simulink model "Full_Model_2"  (R2018b)
settings: Solver=VariableStepAuto  StartTime=0.0  StopTime=.25  RelTol=1e-3
InitFcn:
  | Robot_Body_Constants
values from neighbouring files (symbols this model uses):
  robot_mass = 0.743    [Robot_Body_Constants.m]
  robot_radius = 0.0789    [Robot_Body_Constants.m]
libraries: powerlib x14, simulink x1, peBldcCurrentController x1
settings Model: Creator=Zach  LastModifiedBy=Zach

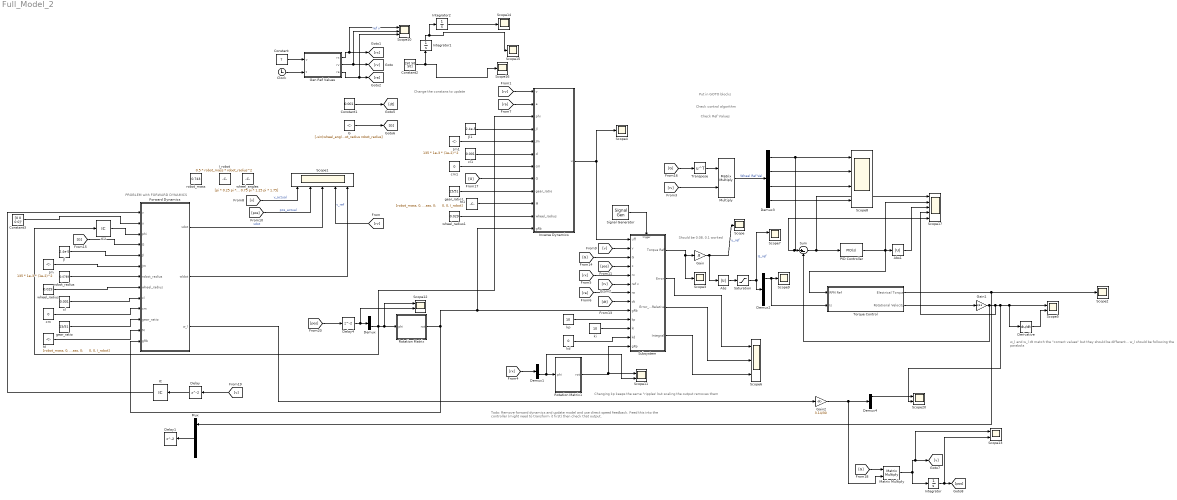
== system Full_Model_2 ==
  note: PROBLEM with FORWARD DYNAMICS
  note: w_l and w_l dt match the "correct values" but they should be different... w_l should be following the parabola
  note: Change the constans to update
  note: Todo: Remove forward dynamics and update model and use direct speed feedback. Feed this into the controller (might need to transform it first) then check that output.
  note: Should be 0.08, 0.1 worked
  note: Changing kp keeps the same "ripples' but scaling the output removes them
  note: Check Ref Values
  note: Check control algorithm
  note: Put in GOTO blocks
  Abs : Abs
  Abs1 : Abs
  Clock : Clock
  Constant : Constant  Value=7
  Constant1 : Constant  Value=0.001
  Constant2 : Constant  Value=[50 50 50]
  Constant3 : Constant  Value=[0 0 0 0]'
  Delay : Delay
  Delay1 : Delay
  Delay4 : Delay
  Demux : Demux  Outputs=3
  Demux1 : Demux  Outputs=3
  Demux2 : Demux
  Demux3 : Demux
  Demux4 : Demux
  Derivative : Derivative
  Forward Dynamics : MATLAB Function  TreatAsAtomicUnit=on
  G : Constant  Value=|
      | [-sin(wheel_angles(1)) -sin(wheel_angles(2)) -sin(wheel_angles(3)) -sin(wheel_angles(4));
      |      cos(wheel_angles(1)) cos(wheel_angles(2)) cos(wheel_angles(3)) cos(wheel_angles(4));
      |      robot_radius robot_radius robot_radius robot_radius]
  Gain : Gain  Gain=.8
  Gain1 : Gain  Gain=1/9.5
  Gain2 : Gain  Gain=3.14/30
  Gen Ref Values : MATLAB Function  TreatAsAtomicUnit=on
  IC : InitialCondition  Value=[0 0 0]'
  IC2 : InitialCondition  Value=0
  I_robot : Constant  Value=0.5 * robot_mass * robot_radius^2
  Integrator : Integrator
  Integrator1 : Integrator
  Integrator2 : Integrator
  Inverse Dynamics : MATLAB Function  TreatAsAtomicUnit=on
  Jl : Constant  Value=2.4e-5
  Jl1 : Constant  Value=2.4e-5
  Jm : Constant  Value=135 * 1e-3 * (1e-2)^2
  Jm1 : Constant  Value=135 * 1e-3 * (1e-2)^2
  M : Constant  Value=|
      | [robot_mass, 0, 0;
      |      0, robot_mass, 0;
      |      0, 0, I_robot]
  M1 : Constant  Value=|
      | [robot_mass, 0, 0;
      |      0, robot_mass, 0;
      |      0, 0, I_robot]
  Matrix Multiply : Product  Multiplication=Matrix(*)
  Multiply : Product  Multiplication=Matrix(*)
  Mux : Mux
  PID Controller : simulink/Continuous/PID Controller  Controller=PID  Form=Parallel  TimeDomain=Continuous-time  SampleTime=-1  IntegratorMethod=Forward Euler  FilterMethod=Forward Euler  ControllerParametersSource=internal  P=10  I=10  D=0  UseFilter=on  N=100  TunerSelectOption=Transfer Function Based (PID Tuner App)  InitialConditionSource=internal  InitialConditionForIntegrator=0  InitialConditionForFilter=0  DifferentiatorICPrevScaledInput=0  ExternalReset=none  TrackingMode=off  Kt=1  LimitOutput=on  UpperSaturationLimit=40  LowerSaturationLimit=-40  LinearizeAsGain=on  AntiWindupMode=none  Kb=1  POutMin=[]  POutMax=[]  IOutMin=[]  IOutMax=[]  DOutMin=[]  DOutMax=[]  NOutMin=[]  NOutMax=[]  SumOutMin=[]  SumOutMax=[]  SaturationOutMin=[]  SaturationOutMax=[]  PParamMin=[]  PParamMax=[]  IParamMin=[]  IParamMax=[]  DParamMin=[]  DParamMax=[]  NParamMin=[]  NParamMax=[]  KbParamMin=[]  KbParamMax=[]  KtParamMin=[]  KtParamMax=[]  KbOutMin=[]  KbOutMax=[]  KtOutMin=[]  KtOutMax=[]  IntegratorOutMin=[]  IntegratorOutMax=[]  FilterOutMin=[]  FilterOutMax=[]  SumI1OutMin=[]  SumI1OutMax=[]  SumI2OutMin=[]  SumI2OutMax=[]  SumI3OutMin=[]  SumI3OutMax=[]  SumI4OutMin=[]  SumI4OutMax=[]  SumDOutMin=[]  SumDOutMax=[]  DifferentiatorOutMin=[]  DifferentiatorOutMax=[]  FilterDiffOutCoefMin=[]  FilterDiffOutCoefMax=[]  ReciprocalOutMin=[]  ReciprocalOutMax=[]  SumDenOutMin=[]  SumDenOutMax=[]  SumNumOutMin=[]  SumNumOutMax=[]  DivideOutMin=[]  DivideOutMax=[]  IntegratorContinuousStateAttributes=''  IntegratorStateMustResolveToSignalObject=off  IntegratorRTWStateStorageClass=Auto  FilterContinuousStateAttributes=''  FilterStateMustResolveToSignalObject=off  FilterRTWStateStorageClass=Auto  ParallelPVariant=InternalParameters  IdealPVariant=Disabled  IVariant=InternalParameters  DVariant=InternalParameters  IntegratorVariant=Continuous  SatVariant=Enabled  AWVariant=Passthrough  PCopyVariant=Disabled  TRVariant=Disabled  FdbkBlocksVariant=Forward  IdealPFdbkVariant=Disabled  SatFdbkVariant=Disabled  DerivativeFilterVariant=ContFilter  NVariant=InternalParameters  NCopyVariant=Disabled  FilterICVariant=InternalICsFilter  IntegratorICVariant=InternalICs  ExternalResetVariant=Disabled  TRSumVariant=Passthrough  SumFdbkVariant=Disabled  SumVariant=Sum_PID
  Rotation Matrix : MATLAB Function  TreatAsAtomicUnit=on
  Rotation Matrix1 : MATLAB Function  TreatAsAtomicUnit=on
  Saturation : Saturate  UpperLimit=40  LowerLimit=-40
  Scope{,2..4,9,14..16} (8 alike) : Scope
  Scope1 : Scope  NumInputPorts=5
  Scope10 : Scope  NumInputPorts=3
  Scope{5,7,11..13,20} (6 alike) : Scope  NumInputPorts=2
  Scope17 : Scope  NumInputPorts=5
  Scope6 : Scope  NumInputPorts=3
  Scope8 : Scope  NumInputPorts=4
  Signal Generator : SignalGenerator  WaveForm=square  Frequency=300  Units=rad/sec
  Subsystem : Subsystem
  Sum : Sum  Inputs=|+-
  Torque Control : Subsystem
  Transpose : Math  Operator=transpose  SaturateOnIntegerOverflow=on
  cl : Constant  Value=0.001
  cl1 : Constant  Value=0.001
  cm : Constant  Value=0
  cm1 : Constant  Value=0
  gear_ratio : Constant  Value=15/51
  gear_ratio1 : Constant  Value=15/51
  kd : Constant  Value=0
  ki : Constant  Value=10
  kp : Constant  Value=10
  robot_mass : Constant  Value=0.743
  robot_radius : Constant  Value=0.0789
  wheel_angles : Constant  Value=[pi * 0.25 pi * 0.75 pi * 1.25 pi * 1.75]
  wheel_radius : Constant  Value=0.029
  wheel_radius1 : Constant  Value=0.029
  wires:
  Delay4/1 -> Scope12/2, Demux/1
  Delay/1 -> IC/1
  IC2/1 -> Forward Dynamics/3(phi)
  Clock/1 -> Gen Ref Values/2(t)
  cl1/1 -> Inverse Dynamics/6(cl)
  gear_ratio/1 -> Forward Dynamics/11(gear_ratio)
  Jm1/1 -> Inverse Dynamics/5(Jm)
  Jl1/1 -> Inverse Dynamics/4(Jl)
  Jl/1 -> Forward Dynamics/5(Jl)
  gear_ratio1/1 -> Inverse Dynamics/9(gear_ratio)
  Gain/1 -> Scope/1, Abs/1  "u_ref"
  Constant1/1 -> [dt]
  M/1 -> Forward Dynamics/12(M)
  Constant/1 -> Gen Ref Values/1(v)
  Rotation Matrix/1(rot) -> Forward Dynamics/13(gRb), Inverse Dynamics/12(gRb), Subsystem/9(gRb)
  Torque Control/1(Electrical Torque) -> Mux/1, Scope2/1
  wheel_radius1/1 -> Inverse Dynamics/11(wheel_radius)
  G/1 -> [G]
  IC/1 -> Forward Dynamics/1(v)
  cl/1 -> Forward Dynamics/9(cl)
  Forward Dynamics/1(vdot) -> Scope1/3  "vdot"
  M1/1 -> Inverse Dynamics/10(M)
  robot_radius/1 -> Forward Dynamics/7(robot_radius)
  cm1/1 -> Inverse Dynamics/7(cm)
  wheel_radius/1 -> Forward Dynamics/8(wheel_radius)
  cm/1 -> Forward Dynamics/10(cm)
  Inverse Dynamics/1(u) -> Subsystem/1(uff), Scope4/1
  Jm/1 -> Forward Dynamics/6(Jm)
  Demux3/2 -> Scope8/2
  Demux3/3 -> Scope8/3
  Demux3/4 -> Scope8/4
  Multiply/1 -> Demux3/1  "Wheel Ref Vel"
  Transpose/1 -> Multiply/1
  Subsystem/1(Torque Ref) -> Scope3/1, Gain/1
  kp/1 -> Subsystem/10(kp)
  ki/1 -> Subsystem/11(ki)
  kd/1 -> Subsystem/12(kd)
  Rotation Matrix1/1(rot) -> Scope11/1, Subsystem/13(gRp)
  Subsystem/2(Error) -> Scope6/1
  Subsystem/3(Error_Path_Relative) -> Scope6/2
  Subsystem/4(Integral) -> Scope6/3
  Signal Generator/1 -> Subsystem/Trigger
  [rv] -> Scope1/4  "v_ref"
  [rv] -> Inverse Dynamics/1(v)
  [rv] -> Subsystem/6(ref v)
  [rv] -> Multiply/2
  [rx] -> Demux1/1
  [rx] -> Subsystem/5(rx)
  [ra] -> Subsystem/7(ra)
  [ra] -> Inverse Dynamics/2(a)
  [v] -> Scope1/1  "v_actual"
  [v] -> Subsystem/2(v)
  [pos] -> Scope1/2  "pos_actual"
  [pos] -> Subsystem/4(x)
  [dt] -> Subsystem/8(dt)
  [G] -> Subsystem/3(G)
  [G] -> Forward Dynamics/4(G)
  [G] -> Transpose/1
  [G] -> Inverse Dynamics/8(G)
  Forward Dynamics/2(wldot) -> Scope1/5
  Abs/1 -> Saturation/1
  Demux2/1 -> Torque Control/2(Is), Scope9/1
  Gain1/1 -> Scope20/2, Derivative/1, Scope5/1, Scope17/4, Sum/2
  Demux/3 -> Inverse Dynamics/3(phi), Scope12/1, Rotation Matrix/1(phi), IC2/1
  Demux1/3 -> Scope11/2, Rotation Matrix1/1(phi)
  Saturation/1 -> Demux2/1, Scope7/1  "Is_ref"
  Gain2/1 -> Matrix Multiply/2, Demux4/1
  [G] -> Matrix Multiply/1
  Matrix Multiply/1 -> Integrator/1, Scope13/1, [v]
  Integrator/1 -> Scope13/2, [pos]
  [v] -> Delay/1
  [pos] -> Delay4/1
  Constant2/1 -> Integrator1/1, Scope16/1
  Integrator1/1 -> Scope15/1, Integrator2/1
  Integrator2/1 -> Scope14/1
  PID Controller/1 -> Abs1/1, Torque Control/1(RPM Ref), Scope17/2
  Abs1/1 -> Scope17/3
  Forward Dynamics/3(w_l) -> Gain2/1
  Demux4/1 -> Scope20/1
  Demux3/1 -> Scope8/1, Scope17/5, Sum/1
  Gen Ref Values/2(rv) -> Scope10/2, [rv]  "ref v"
  Gen Ref Values/1(rx) -> Scope10/1, [rx]
  Gen Ref Values/3(ra) -> Scope10/3, [ra]
  Sum/1 -> PID Controller/1, Scope17/1
  Torque Control/2(Rotational Velocity) -> Gain1/1
  Mux/1 -> Delay1/1
  Derivative/1 -> Scope5/2
  Constant3/1 -> Forward Dynamics/2(u)

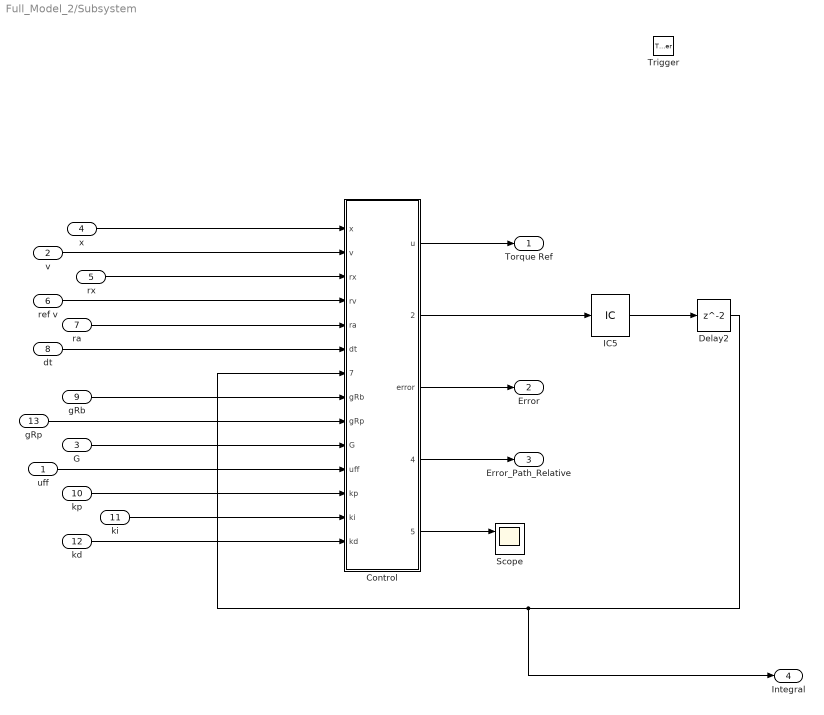
== system Full_Model_2/Subsystem ==
  uff : Inport
  v : Inport  Port=2
  G : Inport  Port=3
  x : Inport  Port=4
  rx : Inport  Port=5
  ref v : Inport  Port=6
  ra : Inport  Port=7
  dt : Inport  Port=8
  gRb : Inport  Port=9
  kp : Inport  Port=10
  ki : Inport  Port=11
  kd : Inport  Port=12
  gRp : Inport  Port=13
  Trigger : TriggerPort  VariantControl=Variant  PortDimensions=1
  Control : MATLAB Function  TreatAsAtomicUnit=on
  Delay2 : Delay
  IC5 : InitialCondition  Value=[0 0 0]
  Scope : Scope  NumInputPorts=2
  Torque Ref : Outport
  Error : Outport  Port=2
  Error_Path_Relative : Outport  Port=3
  Integral : Outport  Port=4
  wires:
  Delay2/1 -> Integral/1, Control/7("integral ")
  uff/1 -> Control/11(uff)
  Control/2(integral) -> IC5/1
  IC5/1 -> Delay2/1
  G/1 -> Control/10(G)
  Control/1(u) -> Torque Ref/1
  rx/1 -> Control/3(rx)
  gRb/1 -> Control/8(gRb)
  ki/1 -> Control/13(ki)
  gRp/1 -> Control/9(gRp)
  kd/1 -> Control/14(kd)
  x/1 -> Control/1(x)
  Control/3(error) -> Error/1
  ra/1 -> Control/5(ra)
  Control/4(error_path_relative) -> Error_Path_Relative/1
  dt/1 -> Control/6(dt)
  ref v/1 -> Control/4(rv)
  v/1 -> Control/2(v)
  kp/1 -> Control/12(kp)
  Control/5(wheel_ref) -> Scope/1

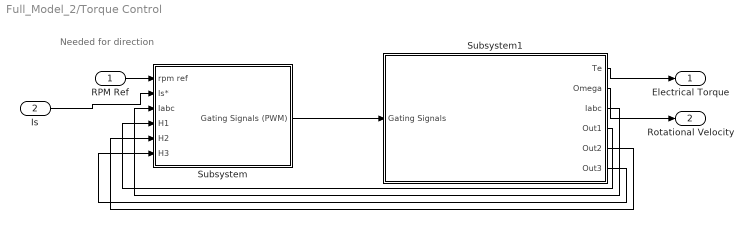
== system Full_Model_2/Torque Control ==
  note: Needed for direction
  RPM Ref : Inport
  Is : Inport  Port=2
  Subsystem : Subsystem
  Subsystem1 : Subsystem
  Electrical Torque : Outport
  Rotational Velocity : Outport  Port=2
  wires:
  Subsystem/1(Gating Signals (PWM)) -> Subsystem1/1(Gating Signals)
  RPM Ref/1 -> Subsystem/1(rpm ref)
  Is/1 -> Subsystem/2(Is*)
  Subsystem1/2(Omega) -> Rotational Velocity/1
  Subsystem1/1(Te) -> Electrical Torque/1
  Subsystem1/3(Iabc) -> Subsystem/3(Iabc)
  Subsystem1/4(Out1) -> Subsystem/4(H1)
  Subsystem1/5(Out2) -> Subsystem/5(H2)
  Subsystem1/6(Out3) -> Subsystem/6(H3)

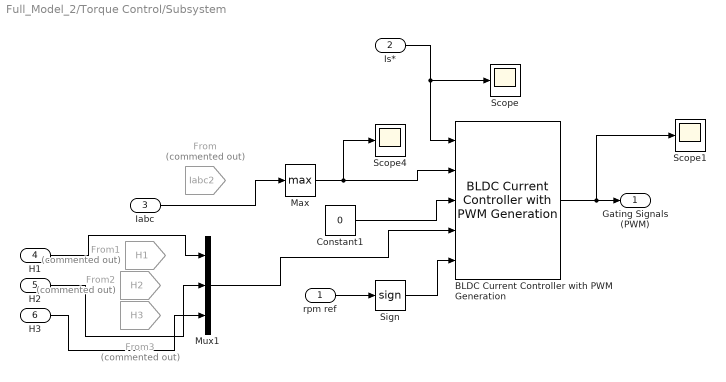
== system Full_Model_2/Torque Control/Subsystem ==
  rpm ref : Inport
  Is* : Inport  Port=2
  Iabc : Inport  Port=3
  H1 : Inport  Port=4
  H2 : Inport  Port=5
  H3 : Inport  Port=6
  BLDC Current Controller with PWM Generation : peBldcCurrentController/BLDC Current Controller with PWM Generation  Kp=40  Ki=10  Kaw=100  Ts=-1  Tsd=0.001  ActZC=off  CarrCount=Up  Tper=.0001  Tfundamental=.00001
  Constant1 : Constant  Value=0
  From : From  Commented=on  GotoTag=Iabc2  TagVisibility=global
  From1 : From  Commented=on  GotoTag=H1  TagVisibility=global
  From2 : From  Commented=on  GotoTag=H2  TagVisibility=global
  From3 : From  Commented=on  GotoTag=H3  TagVisibility=global
  Max : MinMax  Function=max
  Mux1 : Mux  Inputs=3
  Scope : Scope
  Scope1 : Scope
  Scope4 : Scope
  Sign : Signum
  Gating Signals (PWM) : Outport
  wires:
  rpm ref/1 -> Sign/1
  Mux1/1 -> BLDC Current Controller with PWM Generation/4
  Sign/1 -> BLDC Current Controller with PWM Generation/5
  Constant1/1 -> BLDC Current Controller with PWM Generation/3
  Max/1 -> BLDC Current Controller with PWM Generation/2, Scope4/1
  BLDC Current Controller with PWM Generation/1 -> Scope1/1, Gating Signals (PWM)/1
  Is*/1 -> Scope/1, BLDC Current Controller with PWM Generation/1
  Iabc/1 -> Max/1
  H1/1 -> Mux1/1
  H2/1 -> Mux1/2
  H3/1 -> Mux1/3

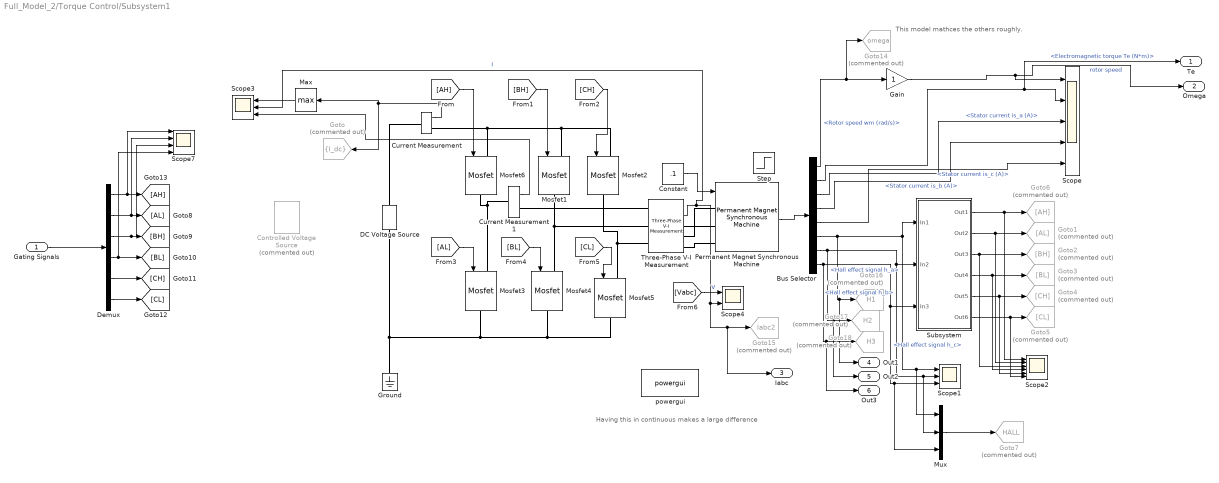
== system Full_Model_2/Torque Control/Subsystem1 ==
  note: This model mathces the others roughly.
  note: Having this in continuous makes a large difference
  Gating Signals : Inport
  Bus Selector : BusSelector  OutputSignals=Rotor speed wm (rad/s),Electromagnetic torque Te (N*m),Stator current is_a (A),Stator current is_b (A),Stator current is_c (A),Hall effect signal h_a,Hall effect signal h_b,Hall effect signal h_c
  Constant : Constant  Value=.1
  Controlled Voltage Source : powerlib/Electrical Sources/Controlled Voltage Source  Commented=on  Initialize=off  Source_Type=DC  Amplitude=24  Phase=0  Frequency=0  Measurements=Voltage
  Current Measurement : powerlib/Measurements/Current Measurement  PhasorSimulation=off  OutputType=Magnitude  PSBequivalent=0
  Current Measurement1 : powerlib/Measurements/Current Measurement  PhasorSimulation=off  OutputType=Complex  PSBequivalent=0
  DC Voltage Source : powerlib/Electrical Sources/DC Voltage Source  Amplitude=24  Measurements=None
  Demux : Demux  Outputs=6
  Gain : Gain
  Goto : Goto  Commented=on  GotoTag=I_dc  TagVisibility=scoped
  Goto1 : Goto  Commented=on  GotoTag=AL
  Goto14 : Goto  Commented=on  GotoTag=omega  TagVisibility=global
  Goto15 : Goto  Commented=on  GotoTag=Iabc2  TagVisibility=global
  Goto16 : Goto  Commented=on  GotoTag=H1  TagVisibility=global
  Goto17 : Goto  Commented=on  GotoTag=H2  TagVisibility=global
  Goto18 : Goto  Commented=on  GotoTag=H3  TagVisibility=global
  Goto2 : Goto  Commented=on  GotoTag=BH
  Goto3 : Goto  Commented=on  GotoTag=BL
  Goto4 : Goto  Commented=on  GotoTag=CH
  Goto5 : Goto  Commented=on  GotoTag=CL
  Goto6 : Goto  Commented=on  GotoTag=AH
  Goto7 : Goto  Commented=on  GotoTag=HALL  TagVisibility=global
  Ground : powerlib/Elements/Ground  LConnTagsString=a
  Max : MinMax  Function=max
  Mosfet{1..6} (6 alike) : powerlib/Power Electronics/Mosfet  Ron=0.1  Lon=0  Rd=0.01  Vfd=0  IC=0  Rs=1e5  Cs=inf  Measurements=off
  Mux : Mux  Inputs=3
  Permanent Magnet Synchronous Machine : powerlib/Machines/Permanent Magnet Synchronous Machine  NbPhases=3  FluxDistribution=Trapezoidal  RotorType=Round  MechanicalLoad=Torque Tm  PresetModel=No  ShowDetailedParameters=on  MeasurementBus=off  Resistance=0.304  Inductance=0.0002315  dqInductances=[8.5e-3,8.5e-3]  La=0.0002315  MachineConstant=Torque Constant (N.m / A_peak)  Flux=0.003258  VoltageCst=5.4588  TorqueCst=0.052128  Flat=120  Mechanical=[1.81e-05 1e-07 8]  PolePairs=4  InitialConditions=[0,0, 0,0]  InitialConditions5ph=[0 0 0 0 0 0]  TsPowergui=0  TsBlock=-1  RefAngle=Aligned with phase A axis (original Park)
      settings: SourceProductName=Simscape Power Systems
  Scope : Scope  NumInputPorts=5
  Scope1 : Scope  NumInputPorts=3
  Scope2 : Scope  NumInputPorts=6
  Scope3 : Scope  NumInputPorts=3
  Scope4 : Scope  NumInputPorts=2
  Scope7 : Scope  NumInputPorts=4
  Step : Step  Time=.1  After=.125  SampleTime=0
  Subsystem : Subsystem
  Three-Phase V-I Measurement : powerlib/Measurements/Three-Phase V-I Measurement  VoltageMeasurement=phase-to-ground  SetLabelV=off  LabelV=Vabc  Vpu=off  VpuLL=off  CurrentMeasurement=yes  SetLabelI=off  LabelI=Iabc  Ipu=off  Pbase=100e6  Vbase=500e3  OutputType=Complex  PhasorSimulation=off  PSBequivalent=0
  powergui : powerlib/powergui  Priority=1  SimulationMode=Continuous  SampleTime=50e-6  frequency=60  Iterations=50  frequencyindice=0  Pbase=100e6  ErrMax=1e-4  UnitsV=kV  UnitsW=MW  buscounter=0  FunctionMessages=off  echomessages=off  EnableUseOfTLC=off  CurrentSourceSwitches=off  DisableSnubberDevices=off  DisableRonSwitches=off  DisableVfSwitches=off  DisplayEquations=off  SolverType=Tustin/Backward Euler (TBE)  Interpol=off  ExternalGateDelay=off  methode=off  Ts=100  x0status=blocks  SPID=on  SwTol=0  HookPort=off  RestoreLinks=warning  ResistiveCurrentMeasurement=off  Frange=[0:2:500]  Ylog=off  Xlog=on  ShowGrid=off  save=off  variable=ZData  structure=0  ZoomFFT=off  StartTime=0.0  cycles=1  DisplayStyle=1  fundamental=60  FreqAxis=off  MaxFrequency=1000  frequencyindicesteady=1  RmsSteady=1  display=off
  Te : Outport
  Omega : Outport  Port=2
  Iabc : Outport  Port=3
  Out1 : Outport  Port=4
  Out2 : Outport  Port=5
  Out3 : Outport  Port=6
  wires:
  [CH] -> Mosfet2/1
  Subsystem/6(Out6) -> Scope2/6, Goto5/1
  Subsystem/2(Out2) -> Scope2/2, Goto1/1
  Bus Selector/8 -> Out3/1, Goto18/1, Mux/3, Scope1/3, Subsystem/3(In3)  "<Hall effect signal h_c>"
  Subsystem/1(Out1) -> Scope2/1, Goto6/1
  Subsystem/3(Out3) -> Scope2/3, Goto2/1
  Bus Selector/2 -> Te/1, Scope/2  "<Electromagnetic torque Te (N*m)>"
  Subsystem/4(Out4) -> Scope2/4, Goto3/1
  Bus Selector/1 -> Goto14/1, Gain/1  "<Rotor speed wm (rad/s)>"
  Bus Selector/7 -> Out2/1, Goto17/1, Mux/2, Scope1/2, Subsystem/2(In2)  "<Hall effect signal h_b>"
  Mux/1 -> Goto7/1
  [AL] -> Mosfet3/1
  [BL] -> Mosfet4/1
  Bus Selector/6 -> Out1/1, Goto16/1, Subsystem/1(In1), Mux/1, Scope1/1  "<Hall effect signal h_a>"
  Subsystem/5(Out5) -> Scope2/5, Goto4/1
  [CL] -> Mosfet5/1
  Current Measurement/1 -> Max/1, Goto/1
  Bus Selector/3 -> Scope/3  "<Stator current is_a (A)>"
  Permanent Magnet Synchronous Machine/1 -> Bus Selector/1
  [BH] -> Mosfet1/1
  [AH] -> Mosfet6/1
  Bus Selector/4 -> Scope/4  "<Stator current is_b (A)>"
  Gain/1 -> Omega/1, Scope/1  "rotor speed"
  Bus Selector/5 -> Scope/5  "<Stator current is_c (A)>"
  Demux/6 -> [CL]
  Demux/5 -> [CH]
  Demux/4 -> [BL], Scope7/4
  Demux/3 -> Scope7/3, [BH]
  Demux/2 -> Scope7/2, [AL]
  Demux/1 -> Scope7/1, [AH]
  [Vabc] -> Scope4/1  "V"
  Three-Phase V-I Measurement/2 -> Iabc/1, Goto15/1, Scope4/2, Scope3/2  "I"
  Gating Signals/1 -> Demux/1
  Max/1 -> Scope3/1
  Current Measurement1/1 -> Scope3/3
  Constant/1 -> Permanent Magnet Synchronous Machine/1
  connections:
  Mosfet1/RConn1 -- Three-Phase V-I Measurement/LConn2 -- Mosfet4/LConn1
  Mosfet2/RConn1 -- Three-Phase V-I Measurement/LConn3 -- Mosfet5/LConn1
  Mosfet6/RConn1 -- Current Measurement1/LConn1 -- Mosfet3/LConn1
  Mosfet6/LConn1 -- Current Measurement/RConn1 -- Mosfet2/LConn1 -- Mosfet1/LConn1
  Ground/LConn1 -- DC Voltage Source/LConn1 -- Mosfet5/RConn1 -- Mosfet4/RConn1 -- Mosfet3/RConn1
  Three-Phase V-I Measurement/RConn1 -- Permanent Magnet Synchronous Machine/LConn1
  Three-Phase V-I Measurement/RConn2 -- Permanent Magnet Synchronous Machine/LConn2
  Permanent Magnet Synchronous Machine/LConn3 -- Three-Phase V-I Measurement/RConn3
  DC Voltage Source/RConn1 -- Current Measurement/LConn1
  Current Measurement1/RConn1 -- Three-Phase V-I Measurement/LConn1

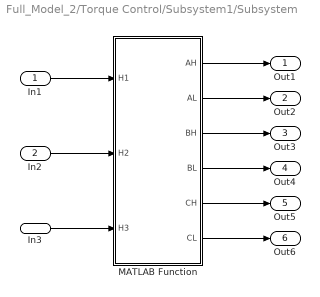
== system Full_Model_2/Torque Control/Subsystem1/Subsystem ==
  In1 : Inport
  In2 : Inport  Port=2
  In3 : Inport  Port=3
  MATLAB Function : MATLAB Function  TreatAsAtomicUnit=on
  Out1 : Outport
  Out2 : Outport  Port=2
  Out3 : Outport  Port=3
  Out4 : Outport  Port=4
  Out5 : Outport  Port=5
  Out6 : Outport  Port=6
  wires:
  In1/1 -> MATLAB Function/1(H1)
  In3/1 -> MATLAB Function/3(H3)
  In2/1 -> MATLAB Function/2(H2)
  MATLAB Function/1(AH) -> Out1/1
  MATLAB Function/2(AL) -> Out2/1
  MATLAB Function/3(BH) -> Out3/1
  MATLAB Function/4(BL) -> Out4/1
  MATLAB Function/6(CL) -> Out6/1
  MATLAB Function/5(CH) -> Out5/1

== matlab function Full_Model_2/Subsystem/Control ==
  data: x input; v input; rx input; rv input; ra input; dt input; u output; integral input; integral output; gRb input; gRp input; G input; uff input; kp input; ki input; kd input; error output; error_path_relative output; wheel_ref output
function [u, integral, error, error_path_relative, wheel_ref] = control(x, v, rx, rv, ra, dt, integral, gRb, gRp, G, uff, kp, ki, kd)
    %gRb = rotation_matrix(x(2));
    %gRp = rotation_matrix(rx(2));
    
    wheel_ref = G' * rv;%inv(gRb) * rv;
    
    error_path_relative = gRp * (rx - x);
    integral = integral + (dt * [1 0 0; 0 1 0; 0 0 1e-2] * error_path_relative);

    Ginv = pinv(G);
    error = gRb' * (rx - x);
    error(3, 1) = error(3, 1) * 0.1;

    derivative = gRb' * (rv - v);
    derivative(3, 1) = derivative(3, 1) * 0.01;

    %uff = inverse_dynamics(rv, ra, x(2));%call inverse_dynamics
    up = kp * Ginv * error;
    ui = ki * Ginv * gRb * gRp' * integral;
    ud = kd * Ginv * derivative;
    
%     uff
%     up
%     ui
%     ud

    u = uff + up + ui + ud;
end

== matlab function Full_Model_2/Torque Control/Subsystem1/Subsystem/MATLAB Function ==
  data: H1 input; AH output; H2 input; H3 input; AL output; BH output; BL output; CH output; CL output
function [AH, AL, BH, BL, CH, CL] = fcn(H1, H2, H3)
% H1 = int16(H1);
% H2 = int16(H2);
% H3 = int16(H3);
H1
H2
H3
AH = 0;
AL = 0;
BH = 0;
BL = 0;
CH = 0;
CL = 0;
%Rember this does not deal with the PWM signal
if (H1(1) == 1 && H2 == 0 && H3 == 0)
    AH = 1;
    AL = 0;
    BH = 0;
    BL = 1;
    CH = 0;
    CL = 0;
elseif (H1(1) == 1 && H2 == 1 && H3 == 0)
    AH = 1;
    AL = 0;
    BH = 0;
    BL = 0;
    CH = 0;
    CL = 1;
elseif (H1(1) == 0 && H2 == 1 && H3 == 0)
    AH = 0;
    AL = 0;
    BH = 1;
    BL = 0;
    CH = 0;
    CL = 1;
elseif (H1(1) == 0 && H2 == 1 && H3 == 1)
    AH = 0;
    AL = 1;
    BH = 1;
    BL = 0;
    CH = 0;
    CL = 0;
elseif (H1(1) == 0 && H2 == 0 && H3 == 1)
    AH = 0;
    AL = 1;
    BH = 0;
    BL = 0;
    CH = 1;
    CL = 0;
elseif (H1(1) == 1 && H2 == 0 && H3 == 1)
    AH = 0;
    AL = 0;
    BH = 0;
    BL = 1;
    CH = 1;
    CL = 0;
end

== matlab function Full_Model_2/Gen Ref Values ==
  data: v input; rx output; t input; rv output; ra output
function [rx, rv, ra] = update_control(v,t)
    rx = [sin(v * t); cos(v * t); v * t];
    rv = v * [cos(v * t); -sin(v * t); v];
    ra = v^2 * [-sin(v * t); -cos(v * t); 0];

%    u = 0.8 * robot_controller.control(pos, vel, rx, rv, ra);
end

== matlab function Full_Model_2/Forward Dynamics ==
  data: v input; u input; vdot output; phi input; G input; Jl input; Jm input; robot_radius input; wheel_radius input; cl input; cm input; gear_ratio input; M input; gRb input; wldot output; w_l output
 function [vdot, wldot, w_l] = forward_dynamics(v, u, phi, G, Jl, Jm, robot_radius, wheel_radius, cl, cm, gear_ratio, M, gRb)
 %To check:
 %Why is it the same when I take output 
    phidot = v(3, 1); %Double check this
    I4 = eye(4);
    GTinv = pinv(G');
    Ginv = pinv(G);
   % gRb = rotation_matrix(phi);
    w_l = G' * gRb' * v / robot_radius; %does not currently match the output of the simulink
    %model rotatinal velocity by an offset that is proportional to speed
    
    Rdot = -phidot * [-sin(phi), -cos(phi), 0; cos(phi), sin(phi), 0; 0, 0, 0];
    RTRdot = phidot * [0 1 0; -1 0 0; 0 0 0];
    
    Z = (((Jm + Jl) / gear_ratio^2) * I4) + (wheel_radius^2/gear_ratio^2) * Ginv * M * GTinv;
    V = ((cm + cl / gear_ratio^2) * I4) + (wheel_radius^2/gear_ratio^2) * Ginv * RTRdot * M * GTinv;
    
    B = pinv(Z)/gear_ratio;
    A = -pinv(Z) * V;
    wldot = A * w_l + B * u;
    
    vdot = Rdot * GTinv * wheel_radius * w_l + gRb * GTinv * wheel_radius * wldot;
end

== matlab function Full_Model_2/Inverse Dynamics ==
  data: v input; u output; a input; phi input; Jl input; Jm input; cl input; cm input; G input; gear_ratio input; M input; wheel_radius input; gRb input
function u = inverse_dynamics(v, a, phi, Jl, Jm, cl, cm, G, gear_ratio, M, wheel_radius, gRb)
    phidot = v(3, 1); %Double check this
    I4 = eye(4);
    GTinv = pinv(G');
    Ginv = pinv(G);
    %gRb = rotation_matrix(phi);
    w_l = G' * gRb' * v / wheel_radius;
    
    Rdot = -phidot * [-sin(phi), -cos(phi), 0; cos(phi), sin(phi), 0; 0, 0, 0];
    RTRdot = phidot * [0 1 0; -1 0 0; 0 0 0];
    
    Z = (((Jm + Jl) / gear_ratio^2) * I4) + (wheel_radius^2/gear_ratio^2) * (Ginv * M) * GTinv;
    v = ((cm + cl / gear_ratio^2) * I4) + (wheel_radius^2/gear_ratio^2) * (Ginv * RTRdot) * GTinv;
    
    wldot = (G' * gRb' / wheel_radius) * (a - Rdot * GTinv * wheel_radius * w_l);
    A = -pinv(Z) * v;
    u = Z * gear_ratio * (wldot - A * w_l);
end

== matlab function Full_Model_2/Rotation Matrix ==
  data: phi input; rot output
function rot = rotation_matrix(phi)
    rot = [cos(phi) -sin(phi) 0; sin(phi) cos(phi) 0; 0 0 1];
end

== matlab function Full_Model_2/Rotation Matrix1 ==
  data: phi input; rot output
function rot = rotation_matrix(phi)
    rot = [cos(phi) -sin(phi) 0; sin(phi) cos(phi) 0; 0 0 1];
end
